simulink model "BasicCANCommunication"  (R2024a)
settings: Solver=VariableStepAuto  StartTime=0.0  StopTime=50  RelTol=1e-3
undefined symbols (not defined in the file): canChannel
libraries: canlib x4, canmsglib x2
settings Model: Creator=The MathWorks, Inc.  LastModifiedBy=prat
settings SolverCC: AlgebraicLoopSolver=TrustRegion  DecoupledContinuousIntegration=on  MinimalZcImpactIntegration=on  MaxZcPerStep=1
settings DataIOCC: ReturnWorkspaceOutputs=off
settings DebuggingCC: UnconnectedInputMsg=warning  UnconnectedOutputMsg=warning  UnconnectedLineMsg=warning  ArithmeticOperatorsInVariantConditions=warning
settings ModelReferenceCC: EnableRefExpFcnMdlSchedulingChecks=on
settings SFSimCC: SimUseLocalCustomCode=off  CustomCodeUndefinedFunction=UseInterfaceOnly
settings RTWCC: RTWUseLocalCustomCode=off  GPUComputeCapability=3.5  DLArmComputeVersion=19.05

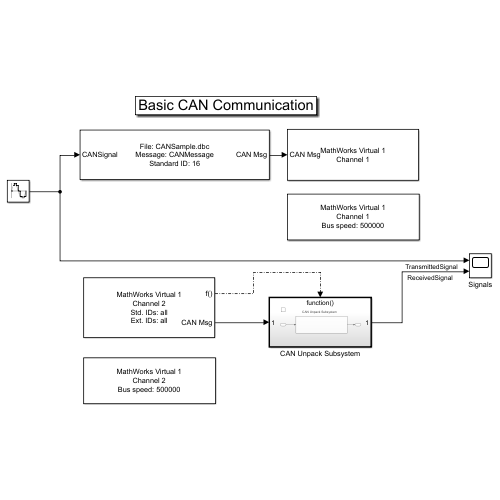
[thumbnail: Simulink's stored preview of the top-level diagram]
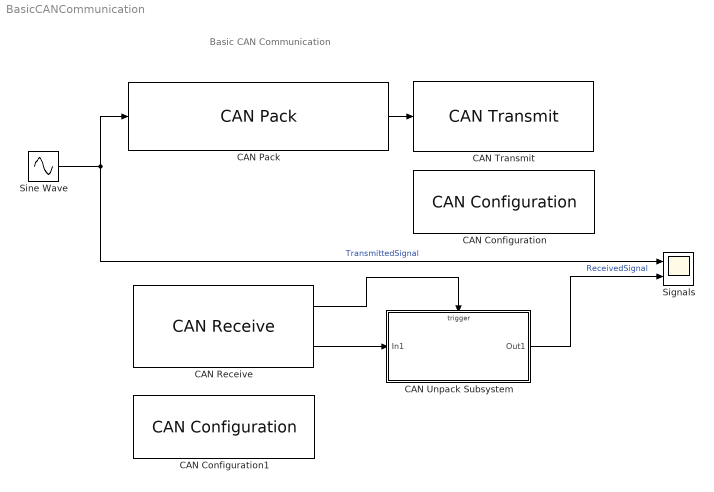
== system BasicCANCommunication ==
  note: Basic CAN Communication
  CAN Configuration : canlib/CAN Configuration  BlockHandle=164.0004  Device=MathWorks Virtual 1 (Channel 1)  DeviceMenu=MathWorks Virtual 1 (Channel 1)  ObjConstructor=canChannel('MathWorks', 'Virtual 1', 1)  BusSpeed=500000  EnableBitParameters=off  AckMode=Normal
  CAN Configuration1 : canlib/CAN Configuration  BlockHandle=165.0004  Device=MathWorks Virtual 1 (Channel 2)  DeviceMenu=MathWorks Virtual 1 (Channel 2)  ObjConstructor=canChannel('MathWorks', 'Virtual 1', 2)  BusSpeed=500000  EnableBitParameters=off  AckMode=Normal
  CAN Pack : canmsglib/CAN Pack  CANdbFile=CANSample.dbc  MsgList=(none)  MsgName=CANMessage  MsgIDType=Standard (11-bit identifier)  MsgIdentifier=16  MsgLength=8  Remote=off  ApplyMinMax=off  BusOutput=on  SignalInfo={'CANSignal','0','64','LE','double','Standard','0','1','0','-1.7e+308','1.7e+308'}
      settings: DataFormat=CANdb specified signals
  CAN Receive : canlib/CAN Receive  BlockHandle=169.0004  Device=MathWorks Virtual 1 (Channel 2)  DeviceMenu=MathWorks Virtual 1 (Channel 2)  ObjConstructor=canChannel('MathWorks', 'Virtual 1', 2)  EnableStandardIDsFilter=off  StdIDsCombo=Allow all  StandardIDs=0  EnableExtendedIDsFilter=off  ExtIDsCombo=Allow all  ExtendedIDs=0  SampleTime=0.01  MsgsPerTimestep=1  InternalFilterUpdateStatus=on  BusOutput=off
  CAN Transmit : canlib/CAN Transmit  BlockHandle=172.0007  Device=MathWorks Virtual 1 (Channel 1)  DeviceMenu=MathWorks Virtual 1 (Channel 1)  ObjConstructor=canChannel('MathWorks', 'Virtual 1', 1)  EnableEventTransmit=off  EnablePeriodicTransmit=off  MessagePeriod=1.000
  CAN Unpack Subsystem : Subsystem  TreatAsAtomicUnit=on
  Signals : Scope  NumInputPorts=2
  Sine Wave : Sin  SampleTime=0.01
  wires:
  Sine Wave/1 -> CAN Pack/1, Signals/1  "TransmittedSignal"
  CAN Pack/1 -> CAN Transmit/1
  CAN Receive/2 -> CAN Unpack Subsystem/1(In1)
  CAN Receive/1 -> CAN Unpack Subsystem/Trigger
  CAN Unpack Subsystem/1(Out1) -> Signals/2  "ReceivedSignal"

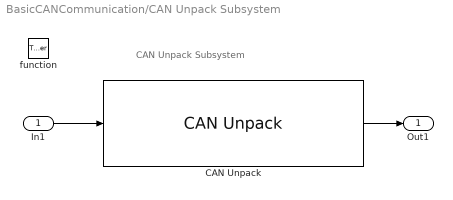
== system BasicCANCommunication/CAN Unpack Subsystem ==
  note: CAN Unpack Subsystem
  In1 : Inport
  function : TriggerPort  TriggerType=function-call  VariantControl=Variant
  CAN Unpack : canmsglib/CAN Unpack  CANdbFile=CANSample.dbc  MsgList=CANMessage  MsgName=CANMessage  MsgIDType=Standard (11-bit identifier)  MsgIdentifier=16  MsgLength=8  SignalInfo={'CANSignal','0','64','LE','double','Standard','0','1','0','-1.7e+308','1.7e+308'}  IDPort=off  TimestampPort=off  ErrorPort=off  RemotePort=off  LengthPort=off  StatusPort=off  ApplyMinMax=off
      settings: DataFormat=CANdb specified signals
  Out1 : Outport  VectorParamsAs1DForOutWhenUnconnected=off
  wires:
  In1/1 -> CAN Unpack/1
  CAN Unpack/1 -> Out1/1
